simulink model "ControlledAngleResponse"  (R2024a)
settings: Solver=VariableStepAuto  StartTime=0.0  StopTime=3  RelTol=1e-3
values from neighbouring files (symbols this model uses):
  K = .65    (= 0.65)    [runControlledForwardResponse.m]    (also in runForwardResponse.m)
  kp = 6.5    [runControlledForwardResponse.m]
  sigma = 11    [runControlledForwardResponse.m]    (also in runForwardResponse.m)
libraries: simulink x1
settings Model: Creator=iankeeffe  LastModifiedBy=lyss5

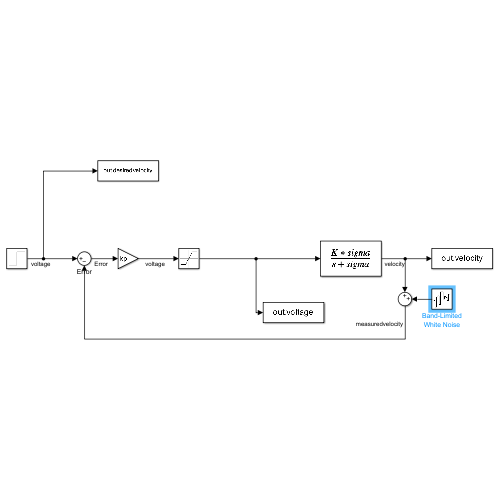
[thumbnail: Simulink's stored preview of the top-level diagram]
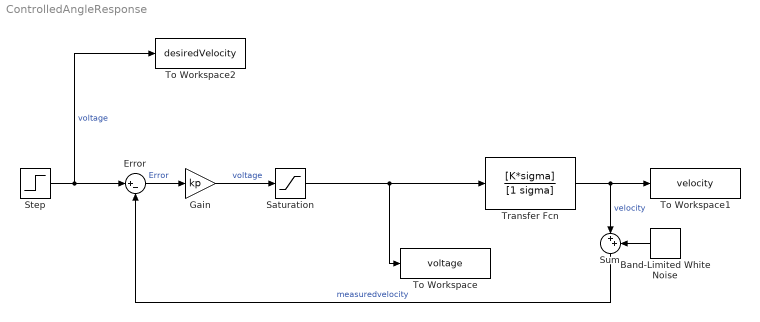
== system ControlledAngleResponse ==
  Band-Limited White Noise : simulink/Sources/Band-Limited White Noise  Cov=[0.0001]  Ts=0.01  seed=[23341]
  Error : Sum  Inputs=|+-
  Gain : Gain  Gain=kp
  Saturation : Saturate  UpperLimit=7.5  LowerLimit=-7.5
  Step : Step  After=.5  SampleTime=0
  Sum : Sum  Inputs=|++
  To Workspace : ToWorkspace  VariableName=voltage  SaveFormat=Timeseries  SampleTime=-1
  To Workspace1 : ToWorkspace  VariableName=velocity  SaveFormat=Timeseries  SampleTime=-1
  To Workspace2 : ToWorkspace  VariableName=desiredVelocity  SaveFormat=Timeseries  SampleTime=-1
  Transfer Fcn : TransferFcn  Numerator=[K*sigma]  Denominator=[1 sigma]
  wires:
  Step/1 -> Error/1, To Workspace2/1  "voltage"
  Transfer Fcn/1 -> Sum/1, To Workspace1/1  "velocity"
  Gain/1 -> Saturation/1  "voltage"
  Error/1 -> Gain/1  "Error"
  Saturation/1 -> To Workspace/1, Transfer Fcn/1
  Band-Limited White Noise/1 -> Sum/2
  Sum/1 -> Error/2  "measuredvelocity"
